simulink model "MS"  (R2022b)
settings: Solver=VariableStepAuto  StartTime=0.0  StopTime=10.0  RelTol=1e-3
values from neighbouring files (symbols this model uses):
  C_ps = 3.0136e+06 * 1e-5    (= 30.136)    [Final_10DOFs_RTHS.m]    (also in ThreeDOFs_CDM_substructure.m = 150.25; structure_2DOFs.m = 0.002)
  K_ps = k9 * 1e-5    (= 1211.4)    [Final_10DOFs_RTHS.m]    (also in ThreeDOFs_CDM_substructure.m = 600; structure_2DOFs.m = 0.012)
  M_ps = m9 * 1e-5    (= 10.7)    [Final_10DOFs_RTHS.m]    (also in ThreeDOFs_CDM_substructure.m = 1; structure_2DOFs.m = 5e-06)
settings Model: Creator=dongxh  LastModifiedBy=dongxh

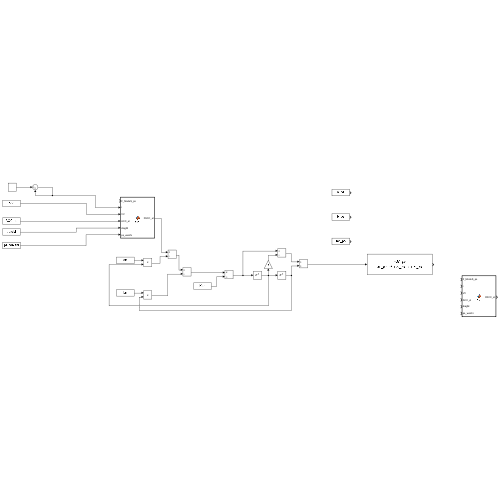
[thumbnail: Simulink's stored preview of the top-level diagram]
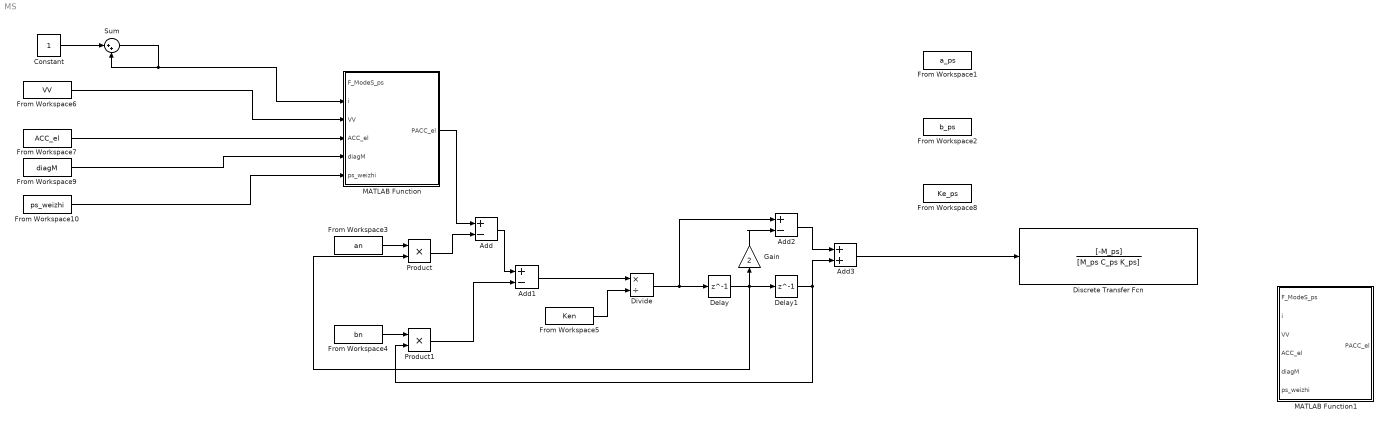
== system MS ==
  Add : Sum  Inputs=+-
  Add1 : Sum  Inputs=+-
  Add2 : Sum  Inputs=+-
  Add3 : Sum
  Constant : Constant
  Delay : Delay  DelayLength=1  InitialCondition=0
  Delay1 : Delay  DelayLength=1  InitialCondition=0
  Discrete Transfer Fcn : DiscreteTransferFcn  Numerator=[-M_ps]  Denominator=[M_ps C_ps K_ps]
  Divide : Product  Inputs=*/
  From Workspace1 : FromWorkspace  VariableName=a_ps
  From Workspace10 : FromWorkspace  VariableName=ps_weizhi
  From Workspace2 : FromWorkspace  VariableName=b_ps
  From Workspace3 : FromWorkspace  VariableName=an
  From Workspace4 : FromWorkspace  VariableName=bn
  From Workspace5 : FromWorkspace  VariableName=Ken
  From Workspace6 : FromWorkspace  VariableName=VV
  From Workspace7 : FromWorkspace  VariableName=ACC_el
  From Workspace8 : FromWorkspace  VariableName=Ke_ps
  From Workspace9 : FromWorkspace  VariableName=diagM
  Gain : Gain  Gain=2
  MATLAB Function : MATLAB Function  TreatAsAtomicUnit=on
  MATLAB Function1 : MATLAB Function  TreatAsAtomicUnit=on
  Product : Product
  Product1 : Product
  Sum : Sum  Inputs=|++
  wires:
  Constant/1 -> Sum/1
  Sum/1 -> MATLAB Function/2(i), Sum/2
  From Workspace6/1 -> MATLAB Function/3(VV)
  From Workspace7/1 -> MATLAB Function/4(ACC_el)
  MATLAB Function/1(PACC_el) -> Add/1
  Product/1 -> Add/2
  Add/1 -> Add1/1
  Product1/1 -> Add1/2
  From Workspace3/1 -> Product/1
  From Workspace4/1 -> Product1/1
  Add1/1 -> Divide/1
  From Workspace5/1 -> Divide/2
  Divide/1 -> Add2/1, Delay/1
  Delay/1 -> Product/2, Gain/1, Delay1/1
  Gain/1 -> Add2/2
  Add2/1 -> Add3/1
  Delay1/1 -> Add3/2, Product1/2
  From Workspace9/1 -> MATLAB Function/5(diagM)
  From Workspace10/1 -> MATLAB Function/6(ps_weizhi)
  Add3/1 -> Discrete Transfer Fcn/1

== matlab function MS/MATLAB Function1 ==
  data: F_ModeS_ps input; PACC_el output; i input; VV input; ACC_el input; diagM input; ps_weizhi input
function PACC_el  = fcn(F_ModeS_ps,i,VV,ACC_el,diagM,ps_weizhi)

end

== matlab function MS/MATLAB Function ==
  data: F_ModeS_ps input; PACC_el output; i input; VV input; ACC_el input; diagM input; ps_weizhi input
function PACC_el  = fcn(F_ModeS_ps,i,VV,ACC_el,diagM,ps_weizhi)
    for ii = 1:order
        PACC_el(ii,i) = VV(:,ii)' * (ACC_el(i, 2) * diagM + F_ModeS_ps(i-1) * ps_weizhi);
    end
end
